simulink model "kinect_sim"  (R2020a)
settings: Solver=FixedStepDiscrete  StartTime=1  StopTime=P.t_end  FixedStep=P.dt  RelTol=1e-3  EnableMultiTasking=on
values from neighbouring files (symbols this model uses):
  P = rmfield(P, 'qbot2_motion_plan')    [kinect_motion_plan.m]
settings Model: ExtModeTrigDuration=10000  Creator=divad  LastModifiedBy=divad
settings SolverCC: PositivePriorityOrder=on
settings DataIOCC: SaveOutput=off  SignalLogging=off  DSMLogging=off  SaveTime=off  ReturnWorkspaceOutputs=off
settings OptimizationCC: LifeSpan=inf
settings DebuggingCC: ArithmeticOperatorsInVariantConditions=warning
settings SFSimCC: SimUseLocalCustomCode=off  CustomCodeUndefinedFunction=UseInterfaceOnly
settings RTWCC: Description=QUARC Win64 Target  SystemTargetFile=quarc_win64.tlc  TemplateMakefile=quarc_default_tmf  RTWUseLocalCustomCode=off
settings CodeAppCC: StateflowObjectComments=on
settings STFCustomTargetCC: TargetPreCompLibLocation=C:\PROGRA~3\QUARC\lib\2020a\win64\release  TargetLangStandard=C99 (ISO)  ConcurrentExecutionCompliant=on  GRTInterface=on  SystemTargetFile=quarc_win64.tlc
settings GRTTargetCC: TargetPreCompLibLocation=C:\PROGRA~3\QUARC\lib\2020a\win64\release  ParMdlRefBuildCompliant=off  CompOptLevelCompliant=off  CombineOutputUpdateFcns=off  MatFileLogging=off  CPPClassGenCompliant=off  GRTInterface=on  UseToolchainInfoCompliant=off  ExtMode=on  ExtModeMexFile=quarc_comm
settings ConfigComp: CovMetricSettings=dswe

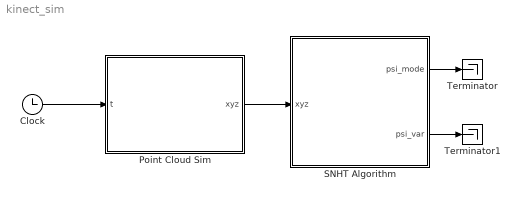
== system kinect_sim ==
  Clock : Clock
  Point Cloud Sim : MATLAB Function  TreatAsAtomicUnit=on
  SNHT Algorithm : Subsystem
  Terminator : Terminator
  Terminator1 : Terminator
  wires:
  Clock/1 -> Point Cloud Sim/1(t)
  Point Cloud Sim/1(xyz) -> SNHT Algorithm/1(xyz)
  SNHT Algorithm/1(psi_mode) -> Terminator/1
  SNHT Algorithm/2(psi_var) -> Terminator1/1

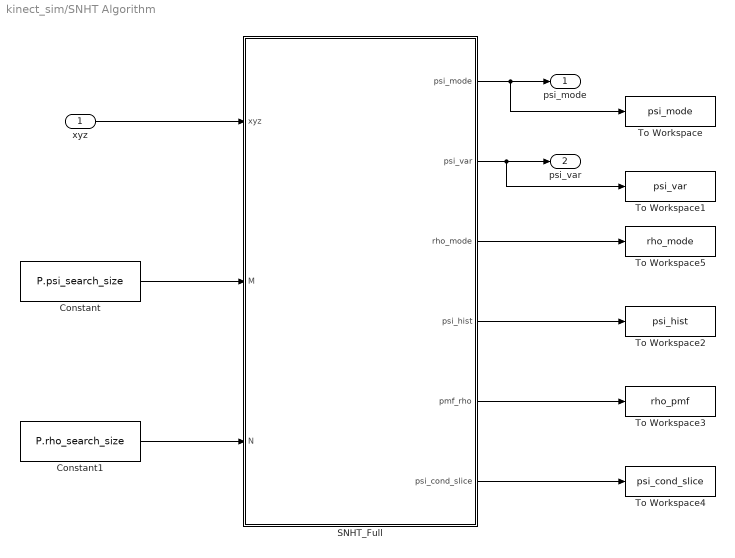
== system kinect_sim/SNHT Algorithm ==
  xyz : Inport
  Constant : Constant  Value=P.psi_search_size
  Constant1 : Constant  Value=P.rho_search_size
  SNHT_Full : MATLAB Function  TreatAsAtomicUnit=on
  To Workspace : ToWorkspace  VariableName=psi_mode  SampleTime=-1
      settings: Save2DSignal=2-D array (concatenate along first dimension)
  To Workspace1 : ToWorkspace  VariableName=psi_var  SampleTime=-1
      settings: Save2DSignal=2-D array (concatenate along first dimension)
  To Workspace2 : ToWorkspace  VariableName=psi_hist  SampleTime=-1
  To Workspace3 : ToWorkspace  VariableName=rho_pmf  SampleTime=-1
      settings: Save2DSignal=2-D array (concatenate along first dimension)
  To Workspace4 : ToWorkspace  VariableName=psi_cond_slice  SampleTime=-1
      settings: Save2DSignal=2-D array (concatenate along first dimension)
  To Workspace5 : ToWorkspace  VariableName=rho_mode  SampleTime=-1
      settings: Save2DSignal=2-D array (concatenate along first dimension)
  psi_mode : Outport
  psi_var : Outport  Port=2
  wires:
  SNHT_Full/2(psi_var) -> To Workspace1/1, psi_var/1
  SNHT_Full/1(psi_mode) -> To Workspace/1, psi_mode/1
  xyz/1 -> SNHT_Full/1(xyz)
  SNHT_Full/6(psi_cond_slice) -> To Workspace4/1
  SNHT_Full/4(psi_hist) -> To Workspace2/1
  SNHT_Full/5(pmf_rho) -> To Workspace3/1
  Constant/1 -> SNHT_Full/2(M)
  Constant1/1 -> SNHT_Full/3(N)
  SNHT_Full/3(rho_mode) -> To Workspace5/1

== matlab function kinect_sim/SNHT Algorithm/SNHT_Full ==
  data: xyz input; M input; N input; psi_mode output; psi_var output; rho_mode output; psi_hist output size=[P.psi_search_size P.rho_search_size]; pmf_rho output; psi_cond_slice output; P parameter
function [psi_mode, psi_var, rho_mode, ...
         psi_hist, pmf_rho, psi_cond_slice] = snht_full(xyz, M, N, P)

%% Call Extrinsic Coder
coder.extrinsic('round');
rho_best_fit = 0;
     
%% Define the Search Space

% Create Psi Bins
psi = P.psi_search;
d_psi = psi(2) - psi(1);

% Define Rho Bins
rho = P.rho_search;
d_rho = rho(2) - rho(1);

% Initialize Accumulator
psi_hist = P.psi_hist_start;
num_votes = 0;
n = 1 : N;

%__________________________________________________________________________
%% Run the SNHT Algorithm

% Iterate all possible psi's for all xyz points on test plane
for k = 1 : length(xyz)
    for ii = 1 : M  % Index psi bins  
        
            % Isolate <x,y> Points
            x = xyz(1, k);
            y = xyz(2, k);
            
            % Transform the <x,y,z> point into the Hough Space
            rho_calc = cos(psi(ii))*x + sin(psi(ii))*y;
            
            % Round Result
            rho_best_fit = double(round(rho_calc, 2));
            
            % Determine which "rho" bin the computation falls into and
            % update the accumulator
            if (rho_best_fit >= rho(1)) && (rho_best_fit <= rho(end))
                
                % Index in the "rho" vector
                rho_mask = rho == rho_best_fit;
                rho_ind = n(rho_mask);
                
                % Update the accumulators
                psi_hist(ii, rho_ind) = psi_hist(ii, rho_ind) + 1;
                
                % Update the number of votes made
                num_votes = num_votes + 1;
                
            end   

    end     
end

%__________________________________________________________________________
%% Calculate the PMF's of psi

%- - - - - - - - - - - - - - - - - - - - - - - - - - - - - - - - - - - - -
% Normailze the Histogram by finding the volume underneath

hist_volume = 0;
for ii = 1 : M      % for each value of psi
    for jj = 1 : N  % for each value of rho
        hist_volume = hist_volume + (d_psi * d_rho * psi_hist(ii,jj));
    end
end

% Normalize the Accumulator
psi_hist = psi_hist ./ hist_volume;

%- - - - - - - - - - - - - - - - - - - - - - - - - - - - - - - - - - - - -
% Find the Marginal PMF of Rho and Normalize

pmf_rho = zeros(1, length(rho));
for jj = 1 : length(rho)
    pmf_rho(jj) = sum(psi_hist(:,jj));
end

% Find the Area under the Rho_PMF
rho_area = 0;
for jj = 1 : N
    rho_area = rho_area + (d_rho * pmf_rho(jj));
end

% Normailze Rho_PMF
pmf_rho = pmf_rho ./ rho_area;

%- - - - - - - - - - - - - - - - - - - - - - - - - - - - - - - - - - - - -
% Find the Conditional Slice of Psi

% Find the mode of Rho
[~, rho_ind] = max(pmf_rho);
rho_mode = rho(rho_ind);

% Extract the slice of Psi where the value of Rho is most probable
psi_cond_slice = psi_hist(:, rho_ind);

% Find the area under the conditional slice of Psi
psi_cond_area = 0;
for ii = 1 : M
    psi_cond_area = psi_cond_area + (d_psi * psi_cond_slice(ii));
end

% Normalize the Conditional Slice
psi_cond_slice = psi_cond_slice ./ psi_cond_area;

%__________________________________________________________________________
%% Extract the Mean and Variance from the PMF's of Psi

% Extract Mode
[~, psi_ind] = max(psi_cond_slice);
psi_mode = psi(psi_ind);

% Extract the Mean
psi_mean = sum(psi .* psi_cond_slice');

% Extract the Variance
psi_var = sum(psi.^2 .* psi_cond_slice') - psi_mean^2; 
psi_var = psi_var / M;

% % Calculate the Std Dev
% if (psi_var <= 0)
%     psi_var = abs(psi_var);
%     neg_flag = 1;
% else
%     neg_flag = 0;
% end
% psi_sigma = sqrt(psi_var);

== matlab function kinect_sim/Point Cloud Sim ==
  data: t input; xyz output; P parameter
function xyz  = point_cloud_sim(t, P)

% Pull out Point Cloud from pre-built Structure
xyz = P.xyz(:,:,t);

% % Return True Psi Values
% front_psi = P.wall_psi(1,t);
% side_psi = P.wall_psi(2,t);
